simulink model "W2P4"  (R2020b)
settings: Solver=VariableStepAuto  StartTime=0.0  StopTime=10.0  RelTol=1e-3
values from neighbouring files (symbols this model uses):
  b = 3.507E-6    [Data.sldd]
  J = 3.228E-6    [Data.sldd]
  K = 0.0275    [Data.sldd]
  Ke = 0.02754    [Data.sldd]
  L = 2.75E-6    [Data.sldd]
  R = 4.0    [Data.sldd]
undefined symbols (not defined in the file or in its folder): Kd, Ki, Kp
settings Model: DataDictionary=Data.sldd  Creator=ASUS  LastModifiedBy=ASUS

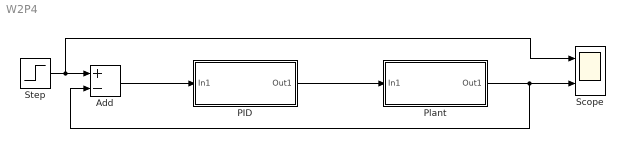
== system W2P4 ==
  Add : Sum  Inputs=+-
  PID : Subsystem
  Plant : Subsystem
  Scope : Scope  NumInputPorts=2
  Step : Step  SampleTime=0
  wires:
  Plant/1(Out1) -> Add/2, Scope/2
  PID/1(Out1) -> Plant/1(In1)
  Step/1 -> Scope/1, Add/1
  Add/1 -> PID/1(In1)

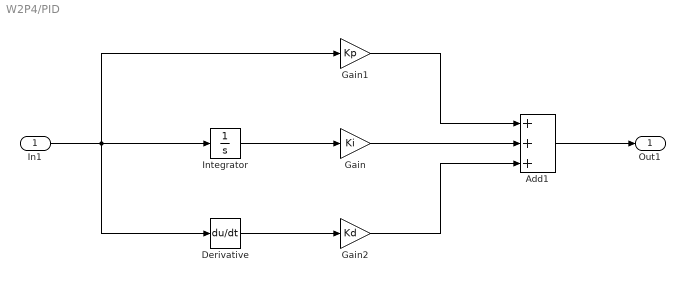
== system W2P4/PID ==
  In1 : Inport
  Add1 : Sum  Inputs=+++
  Derivative : Derivative
  Gain : Gain  Gain=Ki
  Gain1 : Gain  Gain=Kp
  Gain2 : Gain  Gain=Kd
  Integrator : Integrator
  Out1 : Outport
  wires:
  In1/1 -> Gain1/1, Integrator/1, Derivative/1
  Gain2/1 -> Add1/3
  Add1/1 -> Out1/1
  Integrator/1 -> Gain/1
  Derivative/1 -> Gain2/1
  Gain/1 -> Add1/2
  Gain1/1 -> Add1/1

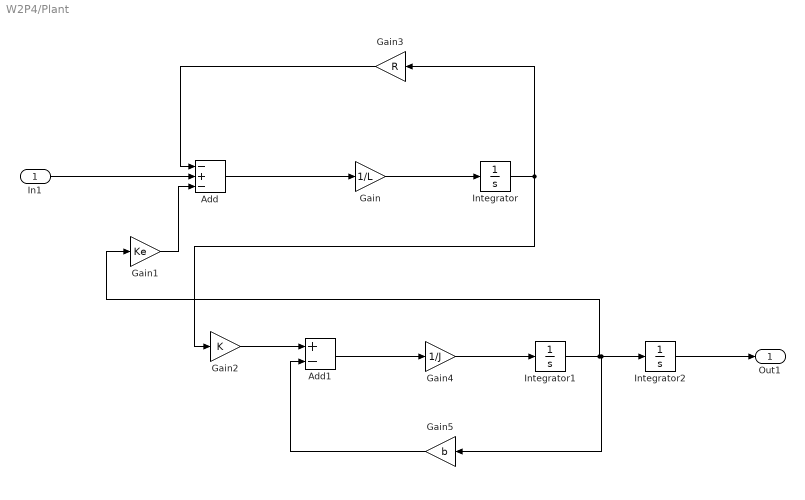
== system W2P4/Plant ==
  In1 : Inport
  Add : Sum  Inputs=-+-
  Add1 : Sum  Inputs=+-
  Gain : Gain  Gain=1/L
  Gain1 : Gain  Gain=Ke
  Gain2 : Gain  Gain=K
  Gain3 : Gain  Gain=R
  Gain4 : Gain  Gain=1/J
  Gain5 : Gain  Gain=b
  Integrator : Integrator
  Integrator1 : Integrator
  Integrator2 : Integrator
  Out1 : Outport
  wires:
  In1/1 -> Add/2
  Add/1 -> Gain/1
  Gain1/1 -> Add/3
  Gain3/1 -> Add/1
  Gain/1 -> Integrator/1
  Integrator/1 -> Gain3/1, Gain2/1
  Gain2/1 -> Add1/1
  Add1/1 -> Gain4/1
  Gain4/1 -> Integrator1/1
  Integrator1/1 -> Gain1/1, Gain5/1, Integrator2/1
  Gain5/1 -> Add1/2
  Integrator2/1 -> Out1/1
